simulink model "math_modeling_simulation"  (R2020a)
settings: Solver=VariableStepAuto  StartTime=0.0  StopTime=100.0  RelTol=1e-3
values from neighbouring files (symbols this model uses):
  b = 0.06    [math_modeling_simulation.m]
  Il = 3    [math_modeling_simulation.m]
  Im = 1    [math_modeling_simulation.m]
  K = 3    [math_modeling_simulation.m]
settings Model: Creator=User  LastModifiedBy=User

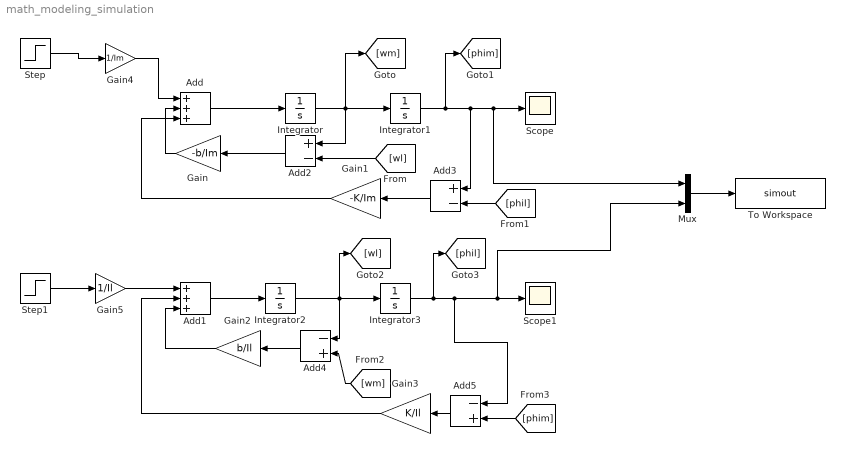
== system math_modeling_simulation ==
  Add : Sum  Inputs=+++
  Add1 : Sum  Inputs=+++
  Add2 : Sum  Inputs=+-
  Add3 : Sum  Inputs=+-
  Add4 : Sum  Inputs=-+
  Add5 : Sum  Inputs=-+
  Gain : Gain  Gain=-b/Im
  Gain1 : Gain  Gain=-K/Im
  Gain2 : Gain  Gain=b/Il
  Gain3 : Gain  Gain=K/Il
  Gain4 : Gain  Gain=1/Im
  Gain5 : Gain  Gain=1/Il
  Integrator{,1..3} (4 alike) : Integrator
  Mux : Mux  Inputs=2
  Scope : Scope
  Scope1 : Scope
  Step : Step  SampleTime=0
  Step1 : Step  SampleTime=0
  To Workspace : ToWorkspace  VariableName=simout  SaveFormat=Timeseries  SampleTime=-1
  wires:
  Integrator/1 -> Add2/1, [wm], Integrator1/1
  Integrator1/1 -> [phim], Add3/1, Mux/1, Scope/1
  Add/1 -> Integrator/1
  Integrator2/1 -> Add4/1, [wl], Integrator3/1
  Integrator3/1 -> [phil], Add5/1, Mux/2, Scope1/1
  Add1/1 -> Integrator2/1
  [wl] -> Add2/2
  Add2/1 -> Gain/1
  Gain/1 -> Add/2
  [phil] -> Add3/2
  Add3/1 -> Gain1/1
  Gain1/1 -> Add/3
  Gain5/1 -> Add1/1
  [wm] -> Add4/2
  Add4/1 -> Gain2/1
  Gain2/1 -> Add1/3
  [phim] -> Add5/2
  Add5/1 -> Gain3/1
  Gain3/1 -> Add1/2
  Mux/1 -> To Workspace/1
  Step/1 -> Gain4/1
  Gain4/1 -> Add/1
  Step1/1 -> Gain5/1
